simulink model "P3_3_2"  (R2018a)
settings: Solver=VariableStepAuto  StartTime=0.0  StopTime=100  RelTol=1e-3
values from neighbouring files (symbols this model uses):
  A_0 = [0 -3.26931291643 0 0.71460251427 0 0 0 0 1 -0.0325743287495 0 -0.000548520916999 ... (64 elements, 8x8)]    [parametros.mat]    (also in twin_rotor_modelo_V1.m = eval(A_0))
  B_0 = [0 0 0 0 0 0 1190.47619048 0 0 0 0 0 ... (16 elements, 8x2)]    [parametros.mat]    (also in twin_rotor_modelo_V1.m = eval(B_0))
  C_0 = [1 0 0 0 0 1 0 0 0 0 0 0 ... (16 elements, 2x8)]    [parametros.mat]    (also in twin_rotor_modelo_V1.m = eval(C_0))
  D_0 = [0  0; 0  0]    [parametros.mat]    (also in twin_rotor_modelo_V1.m = eval(D_0))
  Q = [ ... (first row only)    [ele_cu_erre_para_iterar.m]    (also in elecuerre.m)
  R = [ ... (first row only)    [ele_cu_erre_para_iterar.m]    (also in elecuerre.m; twin_rotor_modelo_V1.m = R2*R1)
  u0 = [11.9668031953 -0.0853053139382]    [parametros.mat]    (also in twin_rotor_modelo_V1.m = [u_p_0;u_t_0])
  x0 = [0.0001 0 0 0 65.3284351132 -0.694344279837 0.788144659543 -0.00372302562915]    [parametros.mat]    (also in twin_rotor_modelo_V1.m = [phi_0; d_phi_0; theta_0; d_theta_0; w_p_0; w_t_0; i_p_0; i_)
undefined symbols (not defined in the file or in its folder): K
libraries: simulink x1
settings Model: Creator=Gonzalo  LastModifiedBy=Gonzalo

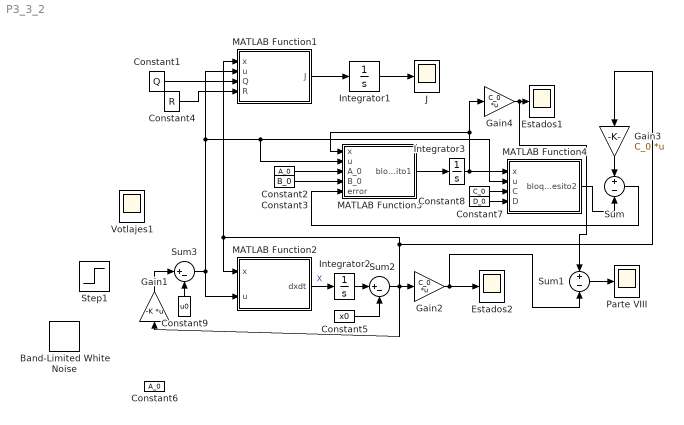
== system P3_3_2 ==
  Band-Limited White Noise : simulink/Sources/Band-Limited White Noise  Cov=[0.0001]  Ts=0.1  seed=[23341]
  Constant1 : Constant  Value=Q
  Constant2 : Constant  Value=A_0
  Constant3 : Constant  Value=B_0
  Constant4 : Constant  Value=R
  Constant5 : Constant  Value=x0
  Constant6 : Constant  Value=A_0
  Constant7 : Constant  Value=C_0
  Constant8 : Constant  Value=D_0
  Constant9 : Constant  Value=u0
  Estados1 : Scope
  Estados2 : Scope
  Gain1 : Gain  Gain=-K  Multiplication=Matrix(K*u)
  Gain2 : Gain  Gain=C_0  Multiplication=Matrix(K*u)
  Gain3 : Gain  Gain=C_0  Multiplication=Matrix(K*u)
  Gain4 : Gain  Gain=C_0  Multiplication=Matrix(K*u)
  Integrator1 : Integrator  InitialCondition=[pi/6 0 0 0 0 0 0 0]
  Integrator2 : Integrator  InitialCondition=[pi/6 0 0 0 0 0 0 0]
  Integrator3 : Integrator  InitialCondition=[pi/6 0 0 0 0 0 0 0]
  J : Scope
  MATLAB Function1 : MATLAB Function  TreatAsAtomicUnit=on
  MATLAB Function2 : MATLAB Function  TreatAsAtomicUnit=on
  MATLAB Function3 : MATLAB Function  TreatAsAtomicUnit=on
  MATLAB Function4 : MATLAB Function  TreatAsAtomicUnit=on
  Parte VIII : Scope
  Step1 : Step  Time=10  Before=u0  After=u0  SampleTime=0
  Sum : Sum  Inputs=+|-
  Sum1 : Sum  Inputs=+|-
  Sum2 : Sum  Inputs=|+-
  Sum3 : Sum  Inputs=|+-
  Votlajes1 : Scope
  wires:
  Sum1/1 -> Parte VIII/1
  Constant7/1 -> MATLAB Function4/3(C)
  Gain3/1 -> Sum/1
  Constant2/1 -> MATLAB Function3/3(A_0)
  Sum/1 -> MATLAB Function3/5(error)
  Constant3/1 -> MATLAB Function3/4(B_0)
  MATLAB Function3/1(bloquesito1) -> Integrator3/1
  Gain4/1 -> Sum1/1, Estados1/1
  MATLAB Function4/1(bloquesito2) -> Sum/2
  Gain2/1 -> Sum1/2, Estados2/1
  Constant1/1 -> MATLAB Function1/3(Q)
  Constant8/1 -> MATLAB Function4/4(D)
  Integrator1/1 -> J/1
  Constant4/1 -> MATLAB Function1/4(R)
  Integrator3/1 -> MATLAB Function4/1(x), Gain4/1, MATLAB Function3/1(x)
  MATLAB Function1/1(J) -> Integrator1/1
  Sum2/1 -> Gain3/1, MATLAB Function2/1(x), MATLAB Function1/1(x), Gain1/1, Gain2/1
  Constant5/1 -> Sum2/2
  Gain1/1 -> Sum3/1
  Constant9/1 -> Sum3/2
  Sum3/1 -> MATLAB Function3/2(u), MATLAB Function4/2(u), MATLAB Function1/2(u), MATLAB Function2/2(u)
  Integrator2/1 -> Sum2/1
  MATLAB Function2/1(dxdt) -> Integrator2/1  "X"

== matlab function P3_3_2/MATLAB Function1 ==
  data: x input; u input; J output; Q input; R input
function J = funcion(x,u,Q,R)
J = x'*Q*x + u'*R*u;

== matlab function P3_3_2/MATLAB Function3 ==
  data: x input; u input; bloquesito1 output; A_0 input; B_0 input; error input
function bloquesito1 = funcion(x,u,A_0,B_0, error)
L =[
    0.0187   -0.0107;
   -0.0006   -0.0012;
   -0.0037    0.0796;
    0.0001    0.0004;
   -0.0000    0.0000;
    0.0000   -0.0000;
    0.0000   -0.0000;
    0.0000    0.0000];
bloquesito1 = A_0*x + B_0*u + L*error

== matlab function P3_3_2/MATLAB Function2 ==
  data: x input; u input; dxdt output
function dxdt = func_f_x(x,u) 
phi = x(1);d_phi = x(2);theta = x(3);d_theta = x(4);w_p = x(5); w_t = x(6); i_p = x(7); i_t = x(8);
u_p = u(1); u_t = u(2);
dxdt = [d_phi;
(((2231553*cos(phi)^2)/4000000 + 6271303914229987/36028797018963968)*((3*d_phi)/250 - (27043227*cos(phi))/20000000 + (3022461*sin(phi))/2500000 + (1256252657407189*d_theta^2*sin(2*phi))/9007199254740992 + (2921964261275593*w_p*abs(w_p))/9223372036854775808))/((1566754414544131*cos(phi)*sin(phi))/9223372036854775808 - (1850992331451507*cos(phi)^2)/9007199254740992 + (3504602316272157*sin(phi)^2)/36893488147419103232 - 4621850957490069/72057594037927936) - (((1027*cos(phi))/25000 + (9189*sin(phi))/200000)*((6466506135038883*w_t*abs(w_t))/368934881474191032320 - (9*d_theta)/5000 + (9*d_phi^2*((9189*cos(phi))/200000 - (1027*sin(phi))/25000))/200 + (1507503188888627*d_phi*d_theta*sin(2*phi))/18014398509481984 + (7304910653188983*w_p*abs(w_p)*sin(phi))/368934881474191032320))/((1566754414544131*cos(phi)*sin(phi))/9223372036854775808 - (1850992331451507*cos(phi)^2)/9007199254740992 + (3504602316272157*sin(phi)^2)/36893488147419103232 - 4621850957490069/72057594037927936);
d_theta;
(((1027*cos(phi))/25000 + (9189*sin(phi))/200000)*((9*d_phi)/2500 - (81129681*cos(phi))/200000000 + (9067383*sin(phi))/25000000 + (1507503188888627*d_theta^2*sin(2*phi))/36028797018963968 + (438294639191339*w_p*abs(w_p))/4611686018427387904))/((1566754414544131*cos(phi)*sin(phi))/9223372036854775808 - (1850992331451507*cos(phi)^2)/9007199254740992 + (3504602316272157*sin(phi)^2)/36893488147419103232 - 4621850957490069/72057594037927936) - ((3177141253833869*w_t*abs(w_t))/73786976294838206464 - (4978621639436999*d_theta)/1125899906842624000 + (4978621639436999*d_phi^2*((9189*cos(phi))/200000 - (1027*sin(phi))/25000))/45035996273704960 + (7406705370233703*d_phi*d_theta*sin(2*phi))/36028797018963968 + (7178136850767151*w_p*abs(w_p)*sin(phi))/147573952589676412928)/((1566754414544131*cos(phi)*sin(phi))/9223372036854775808 - (1850992331451507*cos(phi)^2)/9007199254740992 + (3504602316272157*sin(phi)^2)/36893488147419103232 - 4621850957490069/72057594037927936);
(74600*i_p)/1083 - (300*w_p)/361;
(1492000*i_t)/10609 - (8000*w_t)/10609;
(25000*u_p)/21 - (75000*i_p)/7 - (1865*w_p)/21;
(25000*u_t)/21 - (75000*i_t)/7 - (1865*w_t)/21;
];

== matlab function P3_3_2/MATLAB Function4 ==
  data: x input; u input; bloquesito2 output; C input; D input
function bloquesito2 = funcion(x,u,C,D)
bloquesito2 = C*x + D*u
